simulink model "hw10Q5_model"  (R2021a)
settings: Solver=VariableStepAuto  StartTime=0.0  StopTime=30  RelTol=1e-3
values from neighbouring files (symbols this model uses):
  A = [0 1; 0 0]    [hw10Q5.m]
  B = [0; 1]    [hw10Q5.m]
  C = [1 0]    [hw10Q5.m]
  D = [0]    [hw10Q5.m]
  observer = ss(A + K*C, [B -K], eye(2, 2), zeros(2, 2))    [hw10Q5.m]
libraries: simulink x1
settings Model: Creator=kaiyu  LastModifiedBy=kaiyu

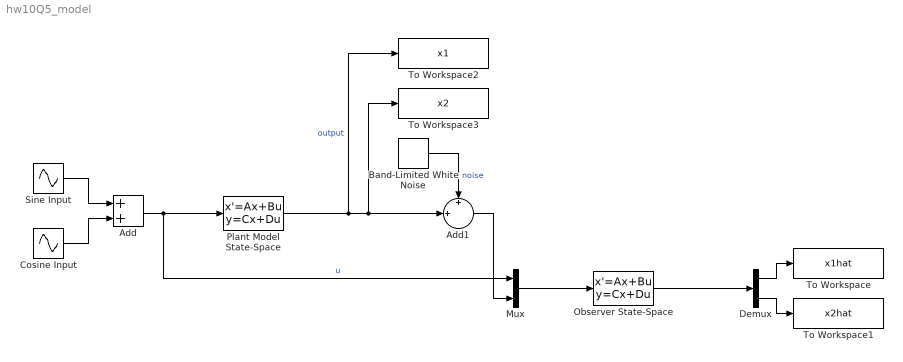
== system hw10Q5_model ==
  Add : Sum
  Add1 : Sum  Inputs=+|+||
  Band-Limited White Noise : simulink/Sources/Band-Limited White Noise  Cov=[0.2]  Ts=0.1  seed=[23341]
  Cosine Input : Sin  Frequency=2  Phase=pi / 2  SampleTime=0
  Demux : Demux  Outputs=2
  Mux : Mux  Inputs=2
  Observer State-Space : StateSpace  A=observer.A  B=observer.B  C=observer.C  D=observer.D  InitialCondition=[3; -2]
  Plant Model State-Space : StateSpace  A=A  B=B  C=C  D=D  InitialCondition=[3; -2]
  Sine Input : Sin  Amplitude=2  SampleTime=0
  To Workspace : ToWorkspace  VariableName=x1hat  SaveFormat=Timeseries  SampleTime=-1
  To Workspace1 : ToWorkspace  VariableName=x2hat  SaveFormat=Timeseries  SampleTime=-1
  To Workspace2 : ToWorkspace  VariableName=x1  SaveFormat=Timeseries  SampleTime=-1
  To Workspace3 : ToWorkspace  VariableName=x2  SaveFormat=Timeseries  SampleTime=-1
  wires:
  Sine Input/1 -> Add/1
  Cosine Input/1 -> Add/2
  Add/1 -> Plant Model State-Space/1, Mux/1  "u"
  Plant Model State-Space/1 -> To Workspace2/1, To Workspace3/1, Add1/2  "output"
  Mux/1 -> Observer State-Space/1
  Band-Limited White Noise/1 -> Add1/1  "noise"
  Add1/1 -> Mux/2
  Observer State-Space/1 -> Demux/1
  Demux/1 -> To Workspace/1
  Demux/2 -> To Workspace1/1
